simulink model "PI_and_I_P"  (R2015a)
settings: Solver=ode45  StartTime=0.0  StopTime=10.0  RelTol=1e-3
values from neighbouring files (symbols this model uses):
  fbon1 = 1    [pi_and_ip.m]
  fbon2 = 0    [pi_and_ip.m]
  Kff = 0    [pi_and_ip.m]
  Kvi = 1    [pi_and_ip.m]
  Kvp = 4    [pi_and_ip.m]
  m = 1    [pi_and_ip.m]    (also in velocity_control_matlab.m = 1;'})
settings Model: Creator=shohei  LastModifiedBy=shohei

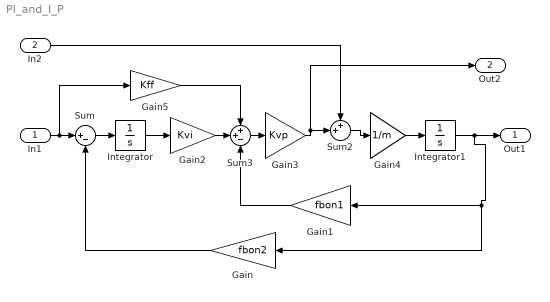
== system PI_and_I_P ==
  In1 : Inport
  In2 : Inport  Port=2
  Gain : Gain  Gain=fbon2
  Gain1 : Gain  Gain=fbon1
  Gain2 : Gain  Gain=Kvi
  Gain3 : Gain  Gain=Kvp
  Gain4 : Gain  Gain=1/m
  Gain5 : Gain  Gain=Kff
  Integrator : Integrator
  Integrator1 : Integrator
  Sum : Sum  Inputs=|+-
  Sum2 : Sum  Inputs=++|
  Sum3 : Sum  Inputs=++-
  Out1 : Outport
  Out2 : Outport  Port=2
  wires:
  In1/1 -> Gain5/1, Sum/1
  Sum/1 -> Integrator/1
  Integrator/1 -> Gain2/1
  Gain2/1 -> Sum3/2
  Gain5/1 -> Sum3/1
  Sum3/1 -> Gain3/1
  Gain3/1 -> Out2/1, Sum2/2
  Sum2/1 -> Gain4/1
  Gain4/1 -> Integrator1/1
  Integrator1/1 -> Gain/1, Gain1/1, Out1/1
  In2/1 -> Sum2/1
  Gain1/1 -> Sum3/3
  Gain/1 -> Sum/2
